simulink model "simulink_learning"  (R2026a)
settings: Solver=VariableStepAuto
libraries: simulink x2
settings Model: Creator=lenovo  LastModifiedBy=lenovo

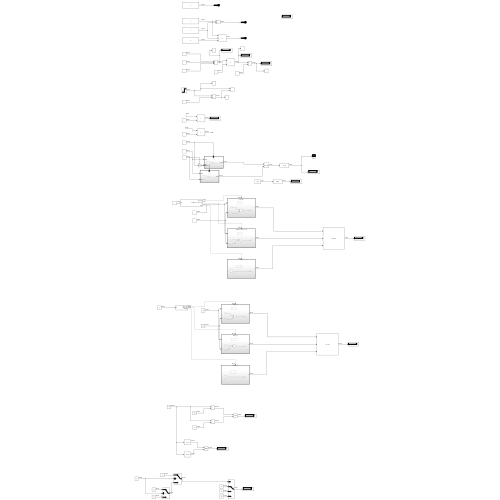
[thumbnail: Simulink's stored preview of the top-level diagram]
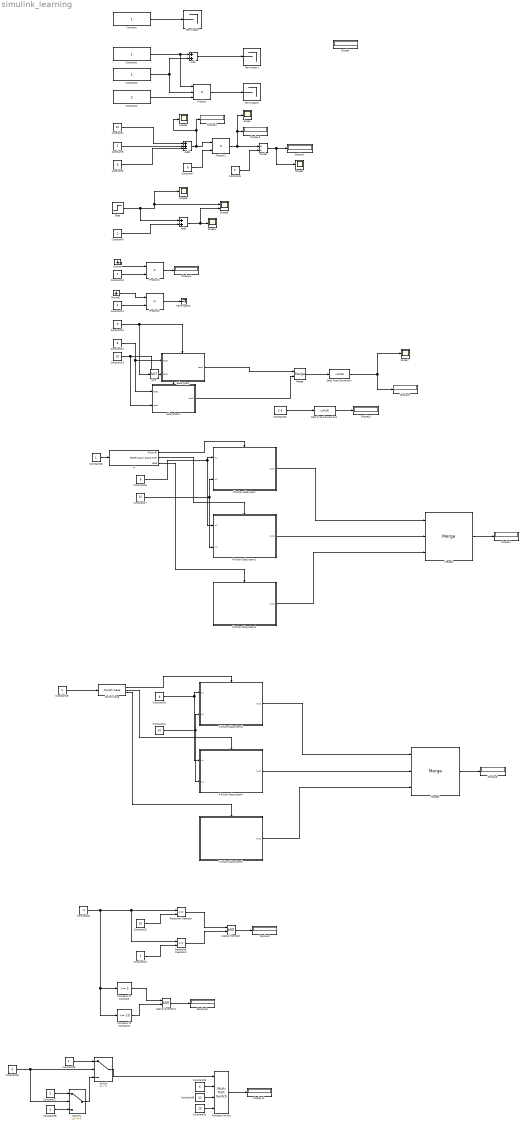
== system simulink_learning ==
  Add : Sum
  Add1 : Sum  Inputs=++-
  Add2 : Sum
  Compare To Constant : simulink/Logic and Bit Operations/Compare To Constant  relop=>=  const=2  OutDataTypeStr=boolean
  Compare To Constant1 : simulink/Logic and Bit Operations/Compare To Constant  relop=<=  const=10  OutDataTypeStr=boolean
  Constant{,1,3,18..19,26} (6 alike) : Constant
  Constant{2,5,8..11,24,27} (8 alike) : Constant  Value=2
  Constant12 : Constant  Value=8
  Constant{4,13,17,21,23} (5 alike) : Constant  Value=10
  Constant14 : Constant  Value=0  OutDataTypeStr=boolean
  Constant15 : Constant  Value=2.6  OutDataTypeStr=single
  Constant16 : Constant  Value=8
  Constant20 : Constant  Value=8
  Constant22 : Constant  Value=4
  Constant25 : Constant  Value=0
  Constant28 : Constant  Value=3
  Constant29 : Constant  Value=6
  Constant30 : Constant  Value=12
  Constant31 : Constant  Value=20
  Constant6 : Constant  Value=6
  Constant7 : Constant  Value=6
  Data Type Conversion : DataTypeConversion  OutDataTypeStr=uint16  SaturateOnIntegerOverflow=off  RndMeth=Floor
  Data Type Conversion1 : DataTypeConversion  OutDataTypeStr=uint16  SaturateOnIntegerOverflow=off  RndMeth=Floor
  Display{,1..11} (12 alike) : Display
  Divide : Product  Inputs=*/
  Ground : Ground
  Ground1 : Ground
  If : If  IfExpression=u1>0  ElseIfExpressions=u1==-1|u1==-6
  If Action Subsystem : Subsystem  TreatAsAtomicUnit=on
  If Action Subsystem1 : Subsystem  TreatAsAtomicUnit=on
  If Action Subsystem2 : Subsystem  TreatAsAtomicUnit=on
  If Action Subsystem3 : Subsystem  TreatAsAtomicUnit=on
  If Action Subsystem4 : Subsystem  TreatAsAtomicUnit=on
  If Action Subsystem5 : Subsystem  TreatAsAtomicUnit=on
  Logical Operator : Logic  AllPortsSameDT=off  OutDataTypeStr=boolean
  Logical Operator1 : Logic  AllPortsSameDT=off  OutDataTypeStr=boolean
  Merge : Merge
  Merge1 : Merge  Inputs=3
  Merge2 : Merge  Inputs=3
  Multiport Switch : MultiPortSwitch  SaturateOnIntegerOverflow=off  InputSameDT=off
  NOT : Logic  Operator=NOT  IconShape=distinctive  AllPortsSameDT=off  OutDataTypeStr=boolean
  Product : Product  Inputs=3
  Product1 : Product
  Product2 : Product
  Product3 : Product
  Relational Operator : RelationalOperator  Operator=<=  OutDataTypeStr=boolean  RndMeth=Simplest  InputSameDT=off
  Relational Operator1 : RelationalOperator  OutDataTypeStr=boolean  RndMeth=Simplest  InputSameDT=off
  Scope{,1..4,7} (6 alike) : Scope
      Scope1 settings: ActiveDisplayYMinimum=5.09472150177857  ActiveDisplayYMaximum=6.9087804586946682
      Scope2 settings: ActiveDisplayYMinimum=10.593890050097921  ActiveDisplayYMaximum=26.264413379467104  DataLoggingVariableName=ScopeData2
      Scope3 settings: ActiveDisplayYMinimum=-20.16976678163514  ActiveDisplayYMaximum=48.939990462720345  DataLoggingVariableName=ScopeData3
      Scope4 settings: ActiveDisplayYMinimum=-5.210931938785329  ActiveDisplayYMaximum=32.502050907679404  DataLoggingVariableName=ScopeData4
      Scope7 settings: ActiveDisplayYMinimum=70  ActiveDisplayYMaximum=90  DataLoggingVariableName=ScopeData7
  Scope5 : Scope  NumInputPorts=2
      settings: ActiveDisplayYMinimum=-22.204611340368309  ActiveDisplayYMaximum=67.04929830985688  DataLoggingVariableName=ScopeData5
  Step : Step  FinalValue=10  SampleTime=0
  Subsystem : Subsystem
  Subsystem1 : Subsystem
  Switch : Switch  Criteria=u2 > Threshold  SaturateOnIntegerOverflow=off  InputSameDT=off
  Switch Case : SwitchCase  CaseConditions={1,2}
  Switch1 : Switch  Criteria=u2 ~= 0  SaturateOnIntegerOverflow=off  InputSameDT=off
  Terminator{,1..3} (4 alike) : Terminator
  wires:
  Constant/1 -> Terminator/1
  Constant1/1 -> Product/1, Add/1
  Constant3/1 -> Product/2, Add/2
  Add/1 -> Terminator1/1
  Product/1 -> Terminator2/1
  Constant2/1 -> Product/3
  Constant4/1 -> Add1/1
  Constant5/1 -> Add1/2
  Constant6/1 -> Add1/3
  Add1/1 -> Scope1/1, Display2/1, Product1/1
  Constant7/1 -> Product1/2
  Product1/1 -> Scope/1, Display3/1, Divide/1
  Constant8/1 -> Divide/2
  Divide/1 -> Scope2/1, Display1/1
  Constant9/1 -> Add2/2
  Step/1 -> Add2/1, Scope5/1, Scope3/1
  Add2/1 -> Scope5/2, Scope4/1
  Ground/1 -> Product2/1
  Constant10/1 -> Product2/2
  Product2/1 -> Display4/1
  Product3/1 -> Terminator3/1
  Ground1/1 -> Product3/1
  Constant11/1 -> Product3/2
  Constant12/1 -> Subsystem1/1(test2), Subsystem/1(test2)
  Constant13/1 -> Subsystem1/2(test1), Subsystem/2(test1)
  Subsystem/1(test3) -> Merge/1
  Constant14/1 -> NOT/1, Subsystem/Enable
  NOT/1 -> Subsystem1/Enable
  Subsystem1/1(test3) -> Merge/2
  Merge/1 -> Data Type Conversion/1
  Data Type Conversion/1 -> Display6/1, Scope7/1
  Constant15/1 -> Data Type Conversion1/1
  Data Type Conversion1/1 -> Display5/1
  If/2 -> If Action Subsystem1/Action
  If/3 -> If Action Subsystem2/Action
  If/1 -> If Action Subsystem/Action
  If Action Subsystem/1(Out1) -> Merge1/1
  If Action Subsystem1/1(Out1) -> Merge1/2
  If Action Subsystem2/1(Out1) -> Merge1/3
  Constant16/1 -> If Action Subsystem/1(In1), If Action Subsystem1/1(In1)
  Constant17/1 -> If Action Subsystem/2(In2), If Action Subsystem1/2(In2)
  Constant18/1 -> If/1
  Merge1/1 -> Display7/1
  Merge2/1 -> Display8/1
  If Action Subsystem3/1(Out1) -> Merge2/1
  If Action Subsystem5/1(Out1) -> Merge2/3
  Constant21/1 -> If Action Subsystem4/2(In2), If Action Subsystem3/2(In2)
  Switch Case/1 -> If Action Subsystem3/Action
  If Action Subsystem4/1(Out1) -> Merge2/2
  Switch Case/3 -> If Action Subsystem5/Action
  Switch Case/2 -> If Action Subsystem4/Action
  Constant20/1 -> If Action Subsystem3/1(In1), If Action Subsystem4/1(In1)
  Constant19/1 -> Switch Case/1
  Constant22/1 -> Compare To Constant1/1, Compare To Constant/1, Relational Operator1/1, Relational Operator/1
  Constant23/1 -> Relational Operator/2
  Constant24/1 -> Relational Operator1/2
  Relational Operator/1 -> Logical Operator/1
  Relational Operator1/1 -> Logical Operator/2
  Logical Operator/1 -> Display9/1
  Compare To Constant/1 -> Logical Operator1/1
  Compare To Constant1/1 -> Logical Operator1/2
  Logical Operator1/1 -> Display10/1
  Constant25/1 -> Switch1/2, Switch/2
  Constant26/1 -> Switch/1
  Constant27/1 -> Switch1/1
  Switch1/1 -> Switch/3
  Constant28/1 -> Switch1/3
  Switch/1 -> Multiport Switch/1
  Constant29/1 -> Multiport Switch/2
  Constant30/1 -> Multiport Switch/3
  Constant31/1 -> Multiport Switch/4
  Multiport Switch/1 -> Display11/1

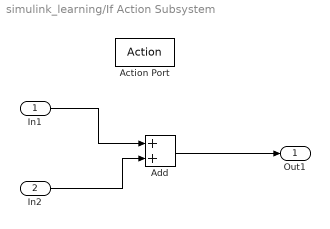
== system simulink_learning/If Action Subsystem ==
  In1 : Inport
  In2 : Inport  Port=2
  Action Port : ActionPort  ActionPortLabel=if(u1>0)
  Add : Sum
  Out1 : Outport
  wires:
  In1/1 -> Add/1
  In2/1 -> Add/2
  Add/1 -> Out1/1

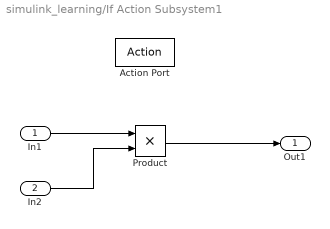
== system simulink_learning/If Action Subsystem1 ==
  In1 : Inport
  In2 : Inport  Port=2
  Action Port : ActionPort  ActionPortLabel=elseif(u1==-1|u1==-6)
  Product : Product
  Out1 : Outport
  wires:
  In1/1 -> Product/1
  In2/1 -> Product/2
  Product/1 -> Out1/1

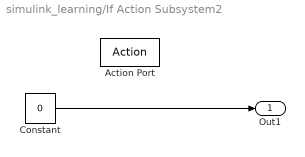
== system simulink_learning/If Action Subsystem2 ==
  Action Port : ActionPort  ActionPortLabel=else
  Constant : Constant  Value=0
  Out1 : Outport
  wires:
  Constant/1 -> Out1/1

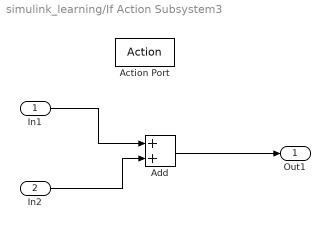
== system simulink_learning/If Action Subsystem3 ==
  In1 : Inport
  In2 : Inport  Port=2
  Action Port : ActionPort  ActionPortLabel=case [ 1 ]:
  Add : Sum
  Out1 : Outport
  wires:
  In1/1 -> Add/1
  In2/1 -> Add/2
  Add/1 -> Out1/1

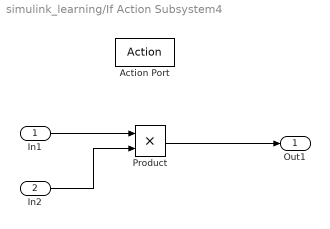
== system simulink_learning/If Action Subsystem4 ==
  In1 : Inport
  In2 : Inport  Port=2
  Action Port : ActionPort  ActionPortLabel=case [ 2 ]:
  Product : Product
  Out1 : Outport
  wires:
  In1/1 -> Product/1
  In2/1 -> Product/2
  Product/1 -> Out1/1

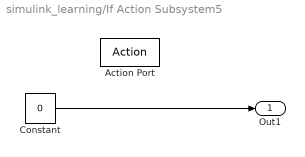
== system simulink_learning/If Action Subsystem5 ==
  Action Port : ActionPort  ActionPortLabel=default:
  Constant : Constant  Value=0
  Out1 : Outport
  wires:
  Constant/1 -> Out1/1

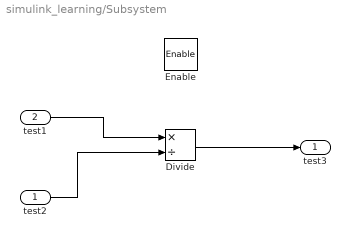
== system simulink_learning/Subsystem ==
  test2 : Inport
  test1 : Inport  Port=2
  Enable : EnablePort
  Divide : Product  Inputs=*/
  test3 : Outport
  wires:
  test1/1 -> Divide/1
  test2/1 -> Divide/2
  Divide/1 -> test3/1

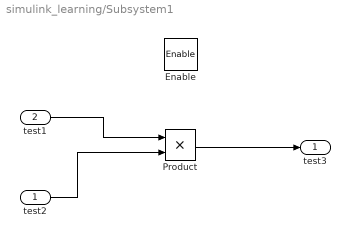
== system simulink_learning/Subsystem1 ==
  test2 : Inport
  test1 : Inport  Port=2
  Enable : EnablePort
  Product : Product
  test3 : Outport
  wires:
  Product/1 -> test3/1
  test2/1 -> Product/2
  test1/1 -> Product/1
